simulink model "m03"  (R2019a)
settings: Solver=ode23  StartTime=0.0  StopTime=30  RelTol=1e-7
settings Model: Creator=wojta  LastModifiedBy=wojta

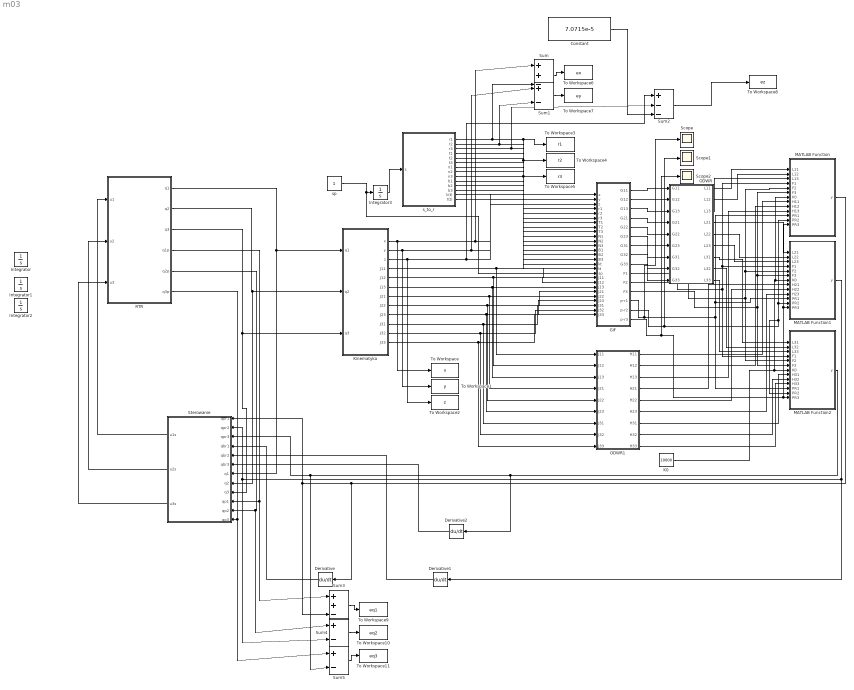
== system m03 ==
  Constant : Constant  Value=7.0715e-5
  Derivative : Derivative
  Derivative1 : Derivative
  Derivative2 : Derivative
  GiF : Subsystem
  Integrator : Integrator  InitialCondition=pi/4
  Integrator1 : Integrator  InitialCondition=0.5
  Integrator2 : Integrator  InitialCondition=-pi/2
  Integrator3 : Integrator
  K0 : Constant  Value=10000
  Kinematyka : Subsystem
  MATLAB Function : MATLAB Function  TreatAsAtomicUnit=on
  MATLAB Function1 : MATLAB Function  TreatAsAtomicUnit=on
  MATLAB Function2 : MATLAB Function  TreatAsAtomicUnit=on
  ODWR : Subsystem
  ODWR1 : Subsystem
  RTR : Subsystem
  Scope : Scope
  Scope1 : Scope
  Scope2 : Scope
  Sterowanie : Subsystem
  Sum : Sum  Inputs=|++-
  Sum1 : Sum  Inputs=|+-
  Sum2 : Sum  Inputs=|+--
  Sum3 : Sum  Inputs=|++-
  Sum4 : Sum  Inputs=|+-
  Sum5 : Sum  Inputs=|+-
  To Workspace : ToWorkspace  VariableName=x  SampleTime=-1
  To Workspace1 : ToWorkspace  VariableName=y  SampleTime=-1
  To Workspace10 : ToWorkspace  VariableName=eq2  SaveFormat=Timeseries  SampleTime=-1
  To Workspace11 : ToWorkspace  VariableName=eq3  SaveFormat=Timeseries  SampleTime=-1
  To Workspace2 : ToWorkspace  VariableName=z  SampleTime=-1
  To Workspace3 : ToWorkspace  VariableName=r1  SampleTime=-1
  To Workspace4 : ToWorkspace  VariableName=r2  SampleTime=-1
  To Workspace5 : ToWorkspace  VariableName=r3  SampleTime=-1
  To Workspace6 : ToWorkspace  VariableName=ex  SaveFormat=Timeseries  SampleTime=-1
  To Workspace7 : ToWorkspace  VariableName=ey  SaveFormat=Timeseries  SampleTime=-1
  To Workspace8 : ToWorkspace  VariableName=ez  SaveFormat=Timeseries  SampleTime=-1
  To Workspace9 : ToWorkspace  VariableName=eq1  SaveFormat=Timeseries  SampleTime=-1
  s_to_r : Subsystem
  sp : Constant
  wires:
  sp/1 -> GiF/18(sp), Integrator3/1
  Integrator3/1 -> s_to_r/1(s)
  Kinematyka/1(x) -> To Workspace/1, Sum/1, GiF/1(x)
  Kinematyka/2(y) -> To Workspace1/1, Sum1/1, GiF/2(y)
  Kinematyka/3(z) -> To Workspace2/1, Sum2/1, GiF/3(z)
  Kinematyka/4(J11) -> ODWR1/1(J11), GiF/19(J11)
  Kinematyka/5(J12) -> ODWR1/2(J12), GiF/20(J12)
  Kinematyka/6(J13) -> ODWR1/3(J13), GiF/21(J13)
  Kinematyka/7(J21) -> ODWR1/4(J21), GiF/22(J21)
  Kinematyka/8(J22) -> ODWR1/5(J22), GiF/23(J22)
  Kinematyka/9(J23) -> ODWR1/6(J23), GiF/24(J23)
  Kinematyka/10(J31) -> ODWR1/7(J31), GiF/25(J31)
  Kinematyka/11(J32) -> ODWR1/8(J32), GiF/26(J32)
  Kinematyka/12(J33) -> ODWR1/9(J33), GiF/27(J33)
  s_to_r/1(r1) -> Sum/3, To Workspace3/1, GiF/4(r1)
  s_to_r/2(r2) -> Sum1/2, To Workspace4/1, GiF/5(r2)
  s_to_r/3(r3) -> Sum2/2, To Workspace5/1, GiF/6(r3)
  s_to_r/4(t1) -> GiF/7(T1)
  s_to_r/5(t2) -> GiF/8(T2)
  s_to_r/6(t3) -> GiF/9(T3)
  s_to_r/7(n1) -> GiF/10(N1)
  s_to_r/8(n2) -> GiF/11(N2)
  s_to_r/9(n3) -> GiF/12(N3)
  s_to_r/10(b1) -> GiF/13(B1)
  s_to_r/11(b2) -> GiF/14(B2)
  s_to_r/12(b3) -> GiF/15(B3)
  s_to_r/13(k(t)) -> GiF/16(kt)
  s_to_r/14(t(t)) -> GiF/17(tt)
  GiF/1(G11) -> ODWR/1(G11)
  GiF/2(G12) -> ODWR/2(G12)
  GiF/3(G13) -> ODWR/3(G13)
  GiF/4(G21) -> ODWR/4(G21)
  GiF/5(G22) -> ODWR/5(G22)
  GiF/6(G23) -> ODWR/6(G23)
  GiF/7(G31) -> ODWR/7(G31)
  GiF/8(G32) -> ODWR/8(G32)
  GiF/9(G33) -> ODWR/9(G33)
  ODWR/1(L11) -> MATLAB Function/1(L11)
  ODWR/2(L12) -> MATLAB Function/2(L12)
  ODWR/3(L13) -> MATLAB Function/3(L13)
  ODWR/4(L21) -> MATLAB Function1/1(L21)
  ODWR/5(L22) -> MATLAB Function1/2(L22)
  ODWR/6(L23) -> MATLAB Function1/3(L23)
  ODWR/7(L31) -> MATLAB Function2/1(L31)
  ODWR/8(L32) -> MATLAB Function2/2(L32)
  ODWR/9(L33) -> MATLAB Function2/3(L33)
  GiF/10(F1) -> MATLAB Function1/4(F1), MATLAB Function/4(F1), MATLAB Function2/4(F1)
  GiF/11(F2) -> MATLAB Function1/5(F2), MATLAB Function/5(F2), MATLAB Function2/5(F2)
  GiF/12(F3) -> MATLAB Function1/6(F3), MATLAB Function/6(F3), MATLAB Function2/6(F3)
  ODWR1/1(H11) -> MATLAB Function/8(H11)
  ODWR1/2(H12) -> MATLAB Function/9(H12)
  ODWR1/3(H13) -> MATLAB Function/10(H13)
  ODWR1/4(H21) -> MATLAB Function1/8(H21)
  ODWR1/5(H22) -> MATLAB Function1/9(H22)
  ODWR1/6(H23) -> MATLAB Function1/10(H23)
  ODWR1/7(H31) -> MATLAB Function2/8(H31)
  ODWR1/8(H32) -> MATLAB Function2/9(H32)
  ODWR1/9(H33) -> MATLAB Function2/10(H33)
  GiF/13(p-r1) -> Scope/1, MATLAB Function2/11(PR1), MATLAB Function1/11(PR1), MATLAB Function/11(PR1)
  GiF/14(p-r2) -> Scope1/1, MATLAB Function2/12(PR2), MATLAB Function1/12(PR2), MATLAB Function/12(PR2)
  GiF/15(p-r3) -> Scope2/1, MATLAB Function/13(PR3), MATLAB Function1/13(PR3), MATLAB Function2/13(PR3)
  K0/1 -> MATLAB Function/7(K0), MATLAB Function1/7(K0), MATLAB Function2/7(K0)
  Sterowanie/2(u2s) -> RTR/2(u2)
  Sterowanie/1(u1s) -> RTR/1(u1)
  Sterowanie/3(u3s) -> RTR/3(u3)
  RTR/1(q1) -> Sterowanie/7(q1), Kinematyka/1(q1)
  RTR/2(q2) -> Sterowanie/8(q2), Kinematyka/2(q2)
  RTR/3(q3) -> Sterowanie/9(q3), Kinematyka/3(q3)
  Derivative/1 -> Sterowanie/4(qbr1)
  Derivative1/1 -> Sterowanie/5(qbr2)
  MATLAB Function2/1(y) -> Derivative2/1, Sum5/2, Sterowanie/3(qpr3)
  Derivative2/1 -> Sterowanie/6(qbr3)
  RTR/4(q1p) -> Sum3/1, Sterowanie/10(qp1)
  RTR/5(q2p) -> Sum4/1, Sterowanie/11(qp2)
  RTR/6(q3p) -> Sum5/1, Sterowanie/12(qp3)
  Sum/1 -> To Workspace6/1
  Sum1/1 -> To Workspace7/1
  Sum2/1 -> To Workspace8/1
  Sum5/1 -> To Workspace11/1
  Sum4/1 -> To Workspace10/1
  Sum3/1 -> To Workspace9/1
  MATLAB Function/1(y) -> Derivative/1, Sum3/3, Sterowanie/1(qpr1)
  MATLAB Function1/1(y) -> Derivative1/1, Sterowanie/2(qpr2), Sum4/2
  Constant/1 -> Sum2/3

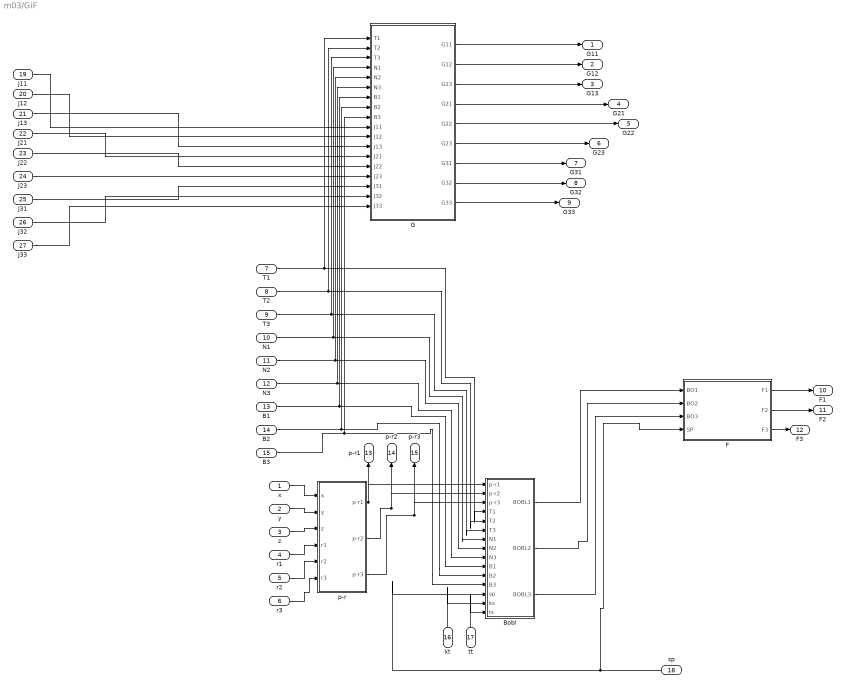
== system m03/GiF ==
  x : Inport
  y : Inport  Port=2
  z : Inport  Port=3
  r1 : Inport  Port=4
  r2 : Inport  Port=5
  r3 : Inport  Port=6
  T1 : Inport  Port=7
  T2 : Inport  Port=8
  T3 : Inport  Port=9
  N1 : Inport  Port=10
  N2 : Inport  Port=11
  N3 : Inport  Port=12
  B1 : Inport  Port=13
  B2 : Inport  Port=14
  B3 : Inport  Port=15
  kt : Inport  Port=16
  tt : Inport  Port=17
  sp : Inport  Port=18
  J11 : Inport  Port=19
  J12 : Inport  Port=20
  J13 : Inport  Port=21
  J21 : Inport  Port=22
  J22 : Inport  Port=23
  J23 : Inport  Port=24
  J31 : Inport  Port=25
  J32 : Inport  Port=26
  J33 : Inport  Port=27
  Bobl : Subsystem
  F : Subsystem
  G : Subsystem
  p-r : Subsystem
  G11 : Outport
  G12 : Outport  Port=2
  G13 : Outport  Port=3
  G21 : Outport  Port=4
  G22 : Outport  Port=5
  G23 : Outport  Port=6
  G31 : Outport  Port=7
  G32 : Outport  Port=8
  G33 : Outport  Port=9
  F1 : Outport  Port=10
  F2 : Outport  Port=11
  F3 : Outport  Port=12
  p-r1 : Outport  Port=13
  p-r2 : Outport  Port=14
  p-r3 : Outport  Port=15
  wires:
  x/1 -> p-r/1(x)
  y/1 -> p-r/2(y)
  z/1 -> p-r/3(z)
  r1/1 -> p-r/4(r1)
  r2/1 -> p-r/5(r2)
  r3/1 -> p-r/6(r3)
  p-r/1(p-r1) -> p-r1/1, Bobl/1(p-r1)
  p-r/2(p-r2) -> p-r2/1, Bobl/2(p-r2)
  p-r/3(p-r3) -> Bobl/3(p-r3), p-r3/1
  T1/1 -> G/1(T1), Bobl/4(T1)
  T2/1 -> G/2(T2), Bobl/5(T2)
  T3/1 -> G/3(T3), Bobl/6(T3)
  N1/1 -> G/4(N1), Bobl/7(N1)
  N2/1 -> G/5(N2), Bobl/8(N2)
  N3/1 -> G/6(N3), Bobl/9(N3)
  B1/1 -> G/7(B1), Bobl/10(B1)
  B2/1 -> G/8(B2), Bobl/11(B2)
  B3/1 -> G/9(B3), Bobl/12(B3)
  sp/1 -> F/4(SP), Bobl/13(sp)
  kt/1 -> Bobl/14(ks)
  tt/1 -> Bobl/15(ts)
  Bobl/1(BOBL1) -> F/1(BO1)
  Bobl/2(BOBL2) -> F/2(BO2)
  Bobl/3(BOBL3) -> F/3(BO3)
  J11/1 -> G/10(J11)
  J12/1 -> G/11(J12)
  J13/1 -> G/12(J13)
  J21/1 -> G/13(J21)
  J22/1 -> G/14(J22)
  J23/1 -> G/15(J23)
  J31/1 -> G/16(J31)
  J32/1 -> G/17(J32)
  J33/1 -> G/18(J33)
  G/1(G11) -> G11/1
  G/2(G12) -> G12/1
  G/3(G13) -> G13/1
  G/4(G21) -> G21/1
  G/5(G22) -> G22/1
  G/6(G23) -> G23/1
  G/7(G31) -> G31/1
  G/8(G32) -> G32/1
  G/9(G33) -> G33/1
  F/1(F1) -> F1/1
  F/2(F2) -> F2/1
  F/3(F3) -> F3/1

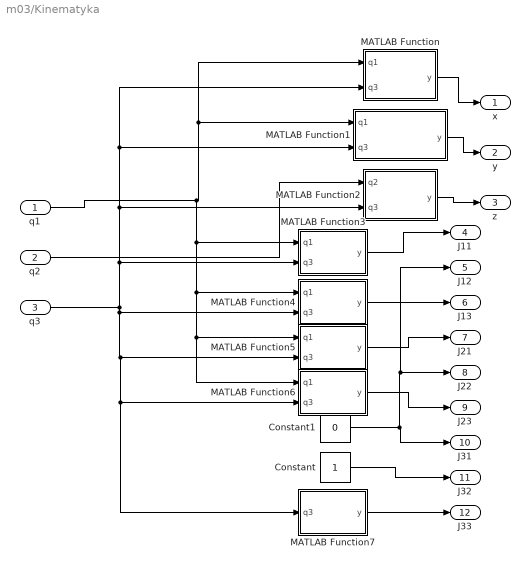
== system m03/Kinematyka ==
  q1 : Inport
  q2 : Inport  Port=2
  q3 : Inport  Port=3
  Constant : Constant
  Constant1 : Constant  Value=0
  MATLAB Function : MATLAB Function  TreatAsAtomicUnit=on
  MATLAB Function1 : MATLAB Function  TreatAsAtomicUnit=on
  MATLAB Function2 : MATLAB Function  TreatAsAtomicUnit=on
  MATLAB Function3 : MATLAB Function  TreatAsAtomicUnit=on
  MATLAB Function4 : MATLAB Function  TreatAsAtomicUnit=on
  MATLAB Function5 : MATLAB Function  TreatAsAtomicUnit=on
  MATLAB Function6 : MATLAB Function  TreatAsAtomicUnit=on
  MATLAB Function7 : MATLAB Function  TreatAsAtomicUnit=on
  x : Outport
  y : Outport  Port=2
  z : Outport  Port=3
  J11 : Outport  Port=4
  J12 : Outport  Port=5
  J13 : Outport  Port=6
  J21 : Outport  Port=7
  J22 : Outport  Port=8
  J23 : Outport  Port=9
  J31 : Outport  Port=10
  J32 : Outport  Port=11
  J33 : Outport  Port=12
  wires:
  MATLAB Function2/1(y) -> z/1
  MATLAB Function1/1(y) -> y/1
  MATLAB Function/1(y) -> x/1
  q1/1 -> MATLAB Function6/1(q1), MATLAB Function5/1(q1), MATLAB Function4/1(q1), MATLAB Function3/1(q1), MATLAB Function/1(q1), MATLAB Function1/1(q1)
  q3/1 -> MATLAB Function3/2(q3), MATLAB Function1/2(q3), MATLAB Function/2(q3), MATLAB Function2/2(q3), MATLAB Function7/1(q3), MATLAB Function6/2(q3), MATLAB Function5/2(q3), MATLAB Function4/2(q3)
  q2/1 -> MATLAB Function2/1(q2)
  MATLAB Function3/1(y) -> J11/1
  MATLAB Function4/1(y) -> J13/1
  MATLAB Function5/1(y) -> J21/1
  MATLAB Function6/1(y) -> J23/1
  MATLAB Function7/1(y) -> J33/1
  Constant/1 -> J32/1
  Constant1/1 -> J12/1, J22/1, J31/1

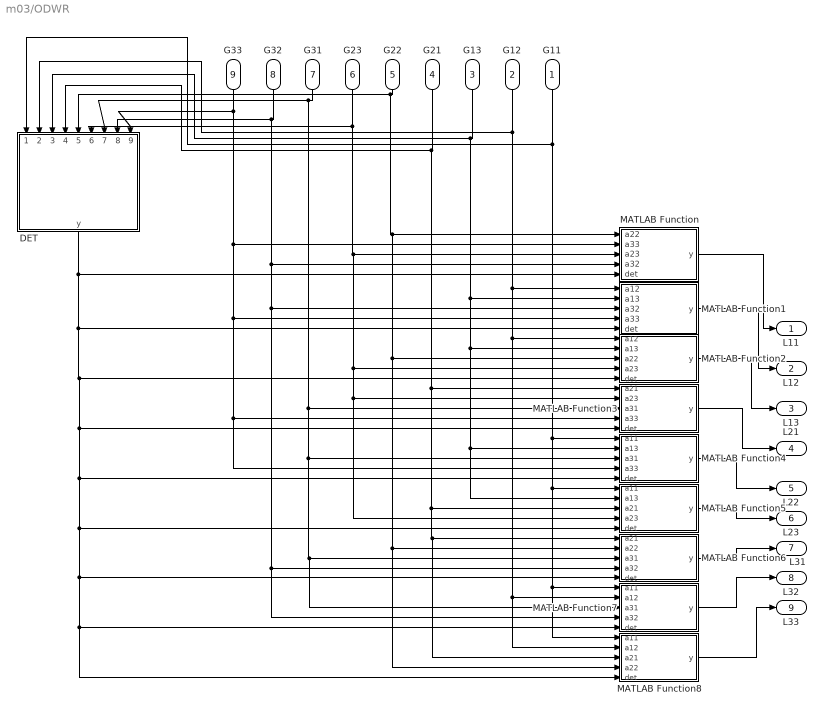
== system m03/ODWR ==
  G11 : Inport
  G12 : Inport  Port=2
  G13 : Inport  Port=3
  G21 : Inport  Port=4
  G22 : Inport  Port=5
  G23 : Inport  Port=6
  G31 : Inport  Port=7
  G32 : Inport  Port=8
  G33 : Inport  Port=9
  DET : MATLAB Function  TreatAsAtomicUnit=on
  MATLAB Function : MATLAB Function  TreatAsAtomicUnit=on
  MATLAB Function1 : MATLAB Function  TreatAsAtomicUnit=on
  MATLAB Function2 : MATLAB Function  TreatAsAtomicUnit=on
  MATLAB Function3 : MATLAB Function  TreatAsAtomicUnit=on
  MATLAB Function4 : MATLAB Function  TreatAsAtomicUnit=on
  MATLAB Function5 : MATLAB Function  TreatAsAtomicUnit=on
  MATLAB Function6 : MATLAB Function  TreatAsAtomicUnit=on
  MATLAB Function7 : MATLAB Function  TreatAsAtomicUnit=on
  MATLAB Function8 : MATLAB Function  TreatAsAtomicUnit=on
  L11 : Outport
  L12 : Outport  Port=2
  L13 : Outport  Port=3
  L21 : Outport  Port=4
  L22 : Outport  Port=5
  L23 : Outport  Port=6
  L31 : Outport  Port=7
  L32 : Outport  Port=8
  L33 : Outport  Port=9
  wires:
  MATLAB Function/1(y) -> L11/1
  MATLAB Function1/1(y) -> L12/1
  MATLAB Function2/1(y) -> L13/1
  MATLAB Function3/1(y) -> L21/1
  MATLAB Function4/1(y) -> L22/1
  MATLAB Function5/1(y) -> L23/1
  MATLAB Function6/1(y) -> L31/1
  MATLAB Function7/1(y) -> L32/1
  MATLAB Function8/1(y) -> L33/1
  G11/1 -> MATLAB Function8/1(a11), MATLAB Function7/1(a11), MATLAB Function5/1(a11), MATLAB Function4/1(a11), DET/1(a11)
  G33/1 -> MATLAB Function4/4(a33), MATLAB Function3/4(a33), MATLAB Function1/4(a33), MATLAB Function/2(a33), DET/9(a33)
  G32/1 -> MATLAB Function7/4(a32), MATLAB Function6/4(a32), MATLAB Function1/3(a32), MATLAB Function/4(a32), DET/8(a32)
  G31/1 -> MATLAB Function7/3(a31), MATLAB Function6/3(a31), MATLAB Function4/3(a31), MATLAB Function3/3(a31), DET/7(a31)
  G23/1 -> MATLAB Function5/4(a23), MATLAB Function3/2(a23), MATLAB Function2/4(a23), MATLAB Function/3(a23), DET/6(a23)
  G22/1 -> MATLAB Function8/4(a22), MATLAB Function6/2(a22), MATLAB Function2/3(a22), MATLAB Function/1(a22), DET/5(a22)
  G21/1 -> MATLAB Function8/3(a21), MATLAB Function6/1(a21), MATLAB Function5/3(a21), MATLAB Function3/1(a21), DET/4(a21)
  G13/1 -> MATLAB Function5/2(a13), MATLAB Function4/2(a13), MATLAB Function2/2(a13), MATLAB Function1/2(a13), DET/3(a13)
  G12/1 -> MATLAB Function8/2(a12), MATLAB Function7/2(a12), MATLAB Function2/1(a12), MATLAB Function1/1(a12), DET/2(a12)
  DET/1(y) -> MATLAB Function8/5(det), MATLAB Function7/5(det), MATLAB Function6/5(det), MATLAB Function5/5(det), MATLAB Function4/5(det), MATLAB Function3/5(det), MATLAB Function2/5(det), MATLAB Function1/5(det), MATLAB Function/5(det)

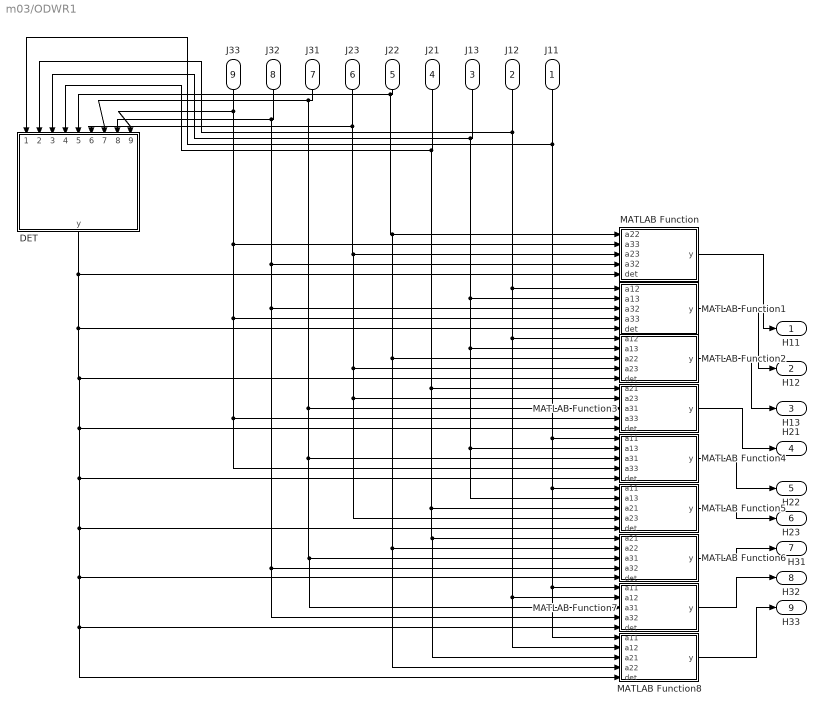
== system m03/ODWR1 ==
  J11 : Inport
  J12 : Inport  Port=2
  J13 : Inport  Port=3
  J21 : Inport  Port=4
  J22 : Inport  Port=5
  J23 : Inport  Port=6
  J31 : Inport  Port=7
  J32 : Inport  Port=8
  J33 : Inport  Port=9
  DET : MATLAB Function  TreatAsAtomicUnit=on
  MATLAB Function : MATLAB Function  TreatAsAtomicUnit=on
  MATLAB Function1 : MATLAB Function  TreatAsAtomicUnit=on
  MATLAB Function2 : MATLAB Function  TreatAsAtomicUnit=on
  MATLAB Function3 : MATLAB Function  TreatAsAtomicUnit=on
  MATLAB Function4 : MATLAB Function  TreatAsAtomicUnit=on
  MATLAB Function5 : MATLAB Function  TreatAsAtomicUnit=on
  MATLAB Function6 : MATLAB Function  TreatAsAtomicUnit=on
  MATLAB Function7 : MATLAB Function  TreatAsAtomicUnit=on
  MATLAB Function8 : MATLAB Function  TreatAsAtomicUnit=on
  H11 : Outport
  H12 : Outport  Port=2
  H13 : Outport  Port=3
  H21 : Outport  Port=4
  H22 : Outport  Port=5
  H23 : Outport  Port=6
  H31 : Outport  Port=7
  H32 : Outport  Port=8
  H33 : Outport  Port=9
  wires:
  MATLAB Function/1(y) -> H11/1
  MATLAB Function1/1(y) -> H12/1
  MATLAB Function2/1(y) -> H13/1
  MATLAB Function3/1(y) -> H21/1
  MATLAB Function4/1(y) -> H22/1
  MATLAB Function5/1(y) -> H23/1
  MATLAB Function6/1(y) -> H31/1
  MATLAB Function7/1(y) -> H32/1
  MATLAB Function8/1(y) -> H33/1
  J11/1 -> MATLAB Function8/1(a11), MATLAB Function7/1(a11), MATLAB Function5/1(a11), MATLAB Function4/1(a11), DET/1(a11)
  J33/1 -> MATLAB Function4/4(a33), MATLAB Function3/4(a33), MATLAB Function1/4(a33), MATLAB Function/2(a33), DET/9(a33)
  J32/1 -> MATLAB Function7/4(a32), MATLAB Function6/4(a32), MATLAB Function1/3(a32), MATLAB Function/4(a32), DET/8(a32)
  J31/1 -> MATLAB Function7/3(a31), MATLAB Function6/3(a31), MATLAB Function4/3(a31), MATLAB Function3/3(a31), DET/7(a31)
  J23/1 -> MATLAB Function5/4(a23), MATLAB Function3/2(a23), MATLAB Function2/4(a23), MATLAB Function/3(a23), DET/6(a23)
  J22/1 -> MATLAB Function8/4(a22), MATLAB Function6/2(a22), MATLAB Function2/3(a22), MATLAB Function/1(a22), DET/5(a22)
  J21/1 -> MATLAB Function8/3(a21), MATLAB Function6/1(a21), MATLAB Function5/3(a21), MATLAB Function3/1(a21), DET/4(a21)
  J13/1 -> MATLAB Function5/2(a13), MATLAB Function4/2(a13), MATLAB Function2/2(a13), MATLAB Function1/2(a13), DET/3(a13)
  J12/1 -> MATLAB Function8/2(a12), MATLAB Function7/2(a12), MATLAB Function2/1(a12), MATLAB Function1/1(a12), DET/2(a12)
  DET/1(y) -> MATLAB Function8/5(det), MATLAB Function7/5(det), MATLAB Function6/5(det), MATLAB Function5/5(det), MATLAB Function4/5(det), MATLAB Function3/5(det), MATLAB Function2/5(det), MATLAB Function1/5(det), MATLAB Function/5(det)

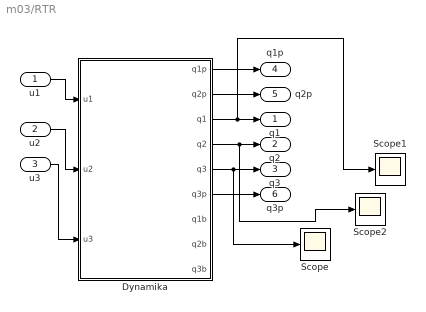
== system m03/RTR ==
  u1 : Inport
  u2 : Inport  Port=2
  u3 : Inport  Port=3
  Dynamika : Subsystem
  Scope : Scope
  Scope1 : Scope
  Scope2 : Scope
  q1 : Outport
  q2 : Outport  Port=2
  q3 : Outport  Port=3
  q1p : Outport  Port=4
  q2p : Outport  Port=5
  q3p : Outport  Port=6
  wires:
  u3/1 -> Dynamika/3(u3)
  u2/1 -> Dynamika/2(u2)
  u1/1 -> Dynamika/1(u1)
  Dynamika/3(q1) -> Scope1/1, q1/1
  Dynamika/4(q2) -> Scope2/1, q2/1
  Dynamika/5(q3) -> Scope/1, q3/1
  Dynamika/1(q1p) -> q1p/1
  Dynamika/2(q2p) -> q2p/1
  Dynamika/6(q3p) -> q3p/1

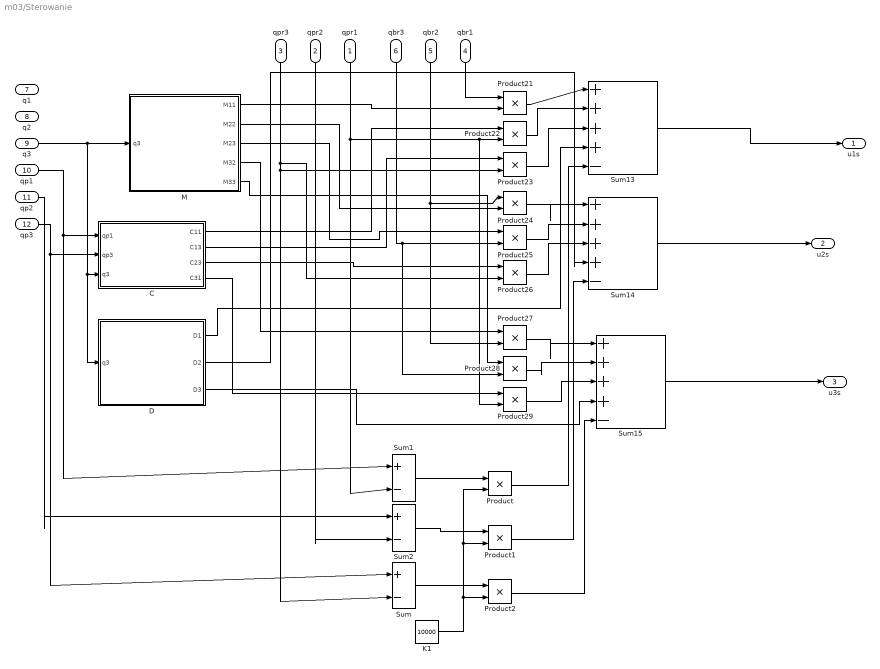
== system m03/Sterowanie ==
  qpr1 : Inport
  qpr2 : Inport  Port=2
  qpr3 : Inport  Port=3
  qbr1 : Inport  Port=4
  qbr2 : Inport  Port=5
  qbr3 : Inport  Port=6
  q1 : Inport  Port=7
  q2 : Inport  Port=8
  q3 : Inport  Port=9
  qp1 : Inport  Port=10
  qp2 : Inport  Port=11
  qp3 : Inport  Port=12
  C : Subsystem
  D : Subsystem
  K1 : Constant  Value=10000
  M : Subsystem
  Product{,1..2,21..29} (12 alike) : Product
  Sum : Sum  Inputs=|+-
  Sum1 : Sum  Inputs=|+-
  Sum13 : Sum  Inputs=|++++-
  Sum14 : Sum  Inputs=|++++-
  Sum15 : Sum  Inputs=|++++-
  Sum2 : Sum  Inputs=|+-
  u1s : Outport
  u2s : Outport  Port=2
  u3s : Outport  Port=3
  wires:
  Sum14/1 -> u2s/1
  Sum15/1 -> u3s/1
  Sum13/1 -> u1s/1
  Product21/1 -> Sum13/1
  Product22/1 -> Sum13/2
  Product23/1 -> Sum13/3
  Product24/1 -> Sum14/1
  Product25/1 -> Sum14/2
  Product26/1 -> Sum14/3
  Product27/1 -> Sum15/1
  Product28/1 -> Sum15/2
  Product29/1 -> Sum15/3
  q3/1 -> D/1(q3), C/3(q3), M/1(q3)
  qp1/1 -> Sum1/1, C/1(qp1)
  qp3/1 -> Sum/1, C/2(qp3)
  qbr1/1 -> Product21/1
  M/1(M11) -> Product21/2
  C/1(C11) -> Product22/1
  C/2(C13) -> Product23/1
  C/3(C23) -> Product26/1
  M/2(M22) -> Product24/2
  M/3(M23) -> Product25/1
  D/1(D1) -> Sum13/4
  D/2(D2) -> Sum14/4
  D/3(D3) -> Sum15/4
  M/4(M32) -> Product27/1
  M/5(M33) -> Product28/1
  C/4(C31) -> Product29/1
  qpr1/1 -> Sum1/2, Product29/2, Product22/2
  qpr3/1 -> Product23/2, Sum/2, Product26/2
  qbr2/1 -> Product27/2, Product24/1
  qbr3/1 -> Product25/2, Product28/2
  qp2/1 -> Sum2/1
  qpr2/1 -> Sum2/2
  K1/1 -> Product/2, Product1/2, Product2/2
  Sum2/1 -> Product1/1
  Sum/1 -> Product2/1
  Sum1/1 -> Product/1
  Product/1 -> Sum13/5
  Product1/1 -> Sum14/5
  Product2/1 -> Sum15/5

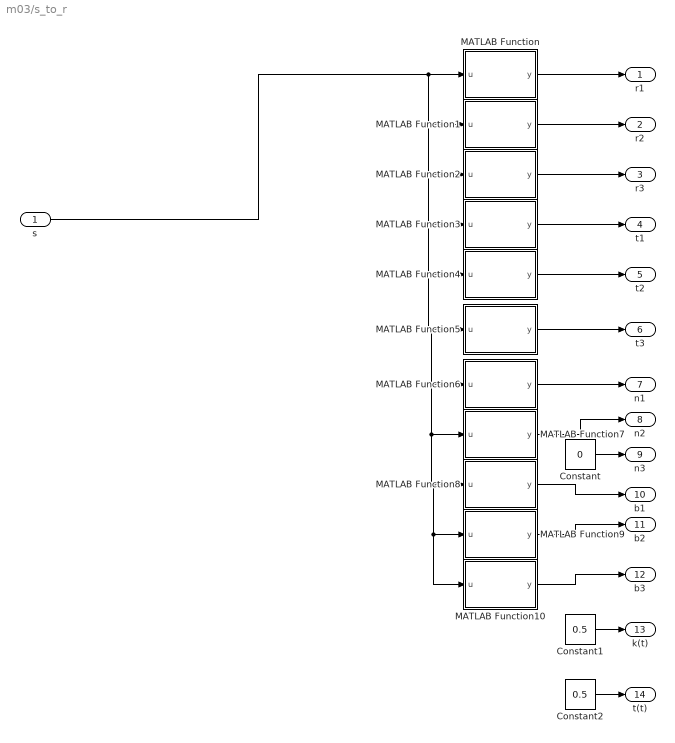
== system m03/s_to_r ==
  s : Inport
  Constant : Constant  Value=0
  Constant1 : Constant  Value=0.5
  Constant2 : Constant  Value=0.5
  MATLAB Function : MATLAB Function  TreatAsAtomicUnit=on
  MATLAB Function1 : MATLAB Function  TreatAsAtomicUnit=on
  MATLAB Function10 : MATLAB Function  TreatAsAtomicUnit=on
  MATLAB Function2 : MATLAB Function  TreatAsAtomicUnit=on
  MATLAB Function3 : MATLAB Function  TreatAsAtomicUnit=on
  MATLAB Function4 : MATLAB Function  TreatAsAtomicUnit=on
  MATLAB Function5 : MATLAB Function  TreatAsAtomicUnit=on
  MATLAB Function6 : MATLAB Function  TreatAsAtomicUnit=on
  MATLAB Function7 : MATLAB Function  TreatAsAtomicUnit=on
  MATLAB Function8 : MATLAB Function  TreatAsAtomicUnit=on
  MATLAB Function9 : MATLAB Function  TreatAsAtomicUnit=on
  r1 : Outport
  r2 : Outport  Port=2
  r3 : Outport  Port=3
  t1 : Outport  Port=4
  t2 : Outport  Port=5
  t3 : Outport  Port=6
  n1 : Outport  Port=7
  n2 : Outport  Port=8
  n3 : Outport  Port=9
  b1 : Outport  Port=10
  b2 : Outport  Port=11
  b3 : Outport  Port=12
  k(t) : Outport  Port=13
  t(t) : Outport  Port=14
  wires:
  MATLAB Function/1(y) -> r1/1
  MATLAB Function1/1(y) -> r2/1
  MATLAB Function2/1(y) -> r3/1
  MATLAB Function3/1(y) -> t1/1
  MATLAB Function4/1(y) -> t2/1
  MATLAB Function5/1(y) -> t3/1
  MATLAB Function6/1(y) -> n1/1
  MATLAB Function7/1(y) -> n2/1
  Constant/1 -> n3/1
  MATLAB Function8/1(y) -> b1/1
  MATLAB Function9/1(y) -> b2/1
  MATLAB Function10/1(y) -> b3/1
  Constant1/1 -> k(t)/1
  Constant2/1 -> t(t)/1
  s/1 -> MATLAB Function10/1(u), MATLAB Function9/1(u), MATLAB Function8/1(u), MATLAB Function7/1(u), MATLAB Function6/1(u), MATLAB Function5/1(u), MATLAB Function4/1(u), MATLAB Function3/1(u), MATLAB Function2/1(u), MATLAB Function1/1(u), MATLAB Function/1(u)

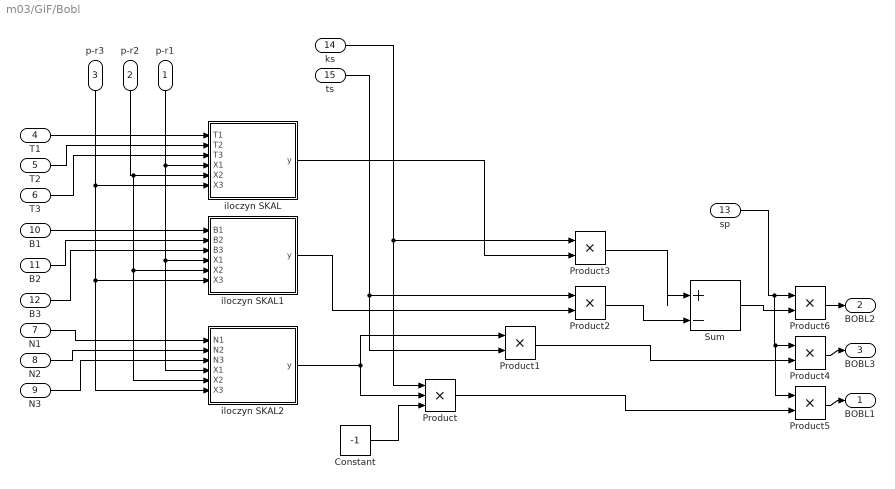
== system m03/GiF/Bobl ==
  p-r1 : Inport
  p-r2 : Inport  Port=2
  p-r3 : Inport  Port=3
  T1 : Inport  Port=4
  T2 : Inport  Port=5
  T3 : Inport  Port=6
  N1 : Inport  Port=7
  N2 : Inport  Port=8
  N3 : Inport  Port=9
  B1 : Inport  Port=10
  B2 : Inport  Port=11
  B3 : Inport  Port=12
  sp : Inport  Port=13
  ks : Inport  Port=14
  ts : Inport  Port=15
  Constant : Constant  Value=-1
  Product : Product  Inputs=3
  Product{1..6} (6 alike) : Product
  Sum : Sum  Inputs=|+-
  iloczyn SKAL : MATLAB Function  TreatAsAtomicUnit=on
  iloczyn SKAL1 : MATLAB Function  TreatAsAtomicUnit=on
  iloczyn SKAL2 : MATLAB Function  TreatAsAtomicUnit=on
  BOBL1 : Outport
  BOBL2 : Outport  Port=2
  BOBL3 : Outport  Port=3
  wires:
  T1/1 -> iloczyn SKAL/1(T1)
  T2/1 -> iloczyn SKAL/2(T2)
  T3/1 -> iloczyn SKAL/3(T3)
  B1/1 -> iloczyn SKAL1/1(B1)
  B2/1 -> iloczyn SKAL1/2(B2)
  B3/1 -> iloczyn SKAL1/3(B3)
  N1/1 -> iloczyn SKAL2/1(N1)
  N2/1 -> iloczyn SKAL2/2(N2)
  N3/1 -> iloczyn SKAL2/3(N3)
  p-r2/1 -> iloczyn SKAL2/5(X2), iloczyn SKAL1/5(X2), iloczyn SKAL/5(X2)
  p-r3/1 -> iloczyn SKAL1/6(X3), iloczyn SKAL2/6(X3), iloczyn SKAL/6(X3)
  p-r1/1 -> iloczyn SKAL2/4(X1), iloczyn SKAL1/4(X1), iloczyn SKAL/4(X1)
  Constant/1 -> Product/3
  iloczyn SKAL2/1(y) -> Product/2, Product1/1
  ks/1 -> Product3/1, Product/1
  ts/1 -> Product2/1, Product1/2
  Product2/1 -> Sum/2
  Product3/1 -> Sum/1
  iloczyn SKAL/1(y) -> Product3/2
  iloczyn SKAL1/1(y) -> Product2/2
  Product6/1 -> BOBL2/1
  Sum/1 -> Product6/2
  Product4/1 -> BOBL3/1
  Product1/1 -> Product4/2
  Product5/1 -> BOBL1/1
  Product/1 -> Product5/2
  sp/1 -> Product5/1, Product4/1, Product6/1

== system m03/GiF/F ==
  BO1 : Inport
  BO2 : Inport  Port=2
  BO3 : Inport  Port=3
  SP : Inport  Port=4
  Sum : Sum  Inputs=|--
  Sum1 : Sum  Inputs=|--
  Sum2 : Sum  Inputs=|--
  F1 : Outport
  F2 : Outport  Port=2
  F3 : Outport  Port=3
  wires:
  BO1/1 -> Sum/1
  BO2/1 -> Sum1/1
  BO3/1 -> Sum2/1
  SP/1 -> Sum2/2, Sum/2, Sum1/2
  Sum/1 -> F1/1
  Sum1/1 -> F2/1
  Sum2/1 -> F3/1

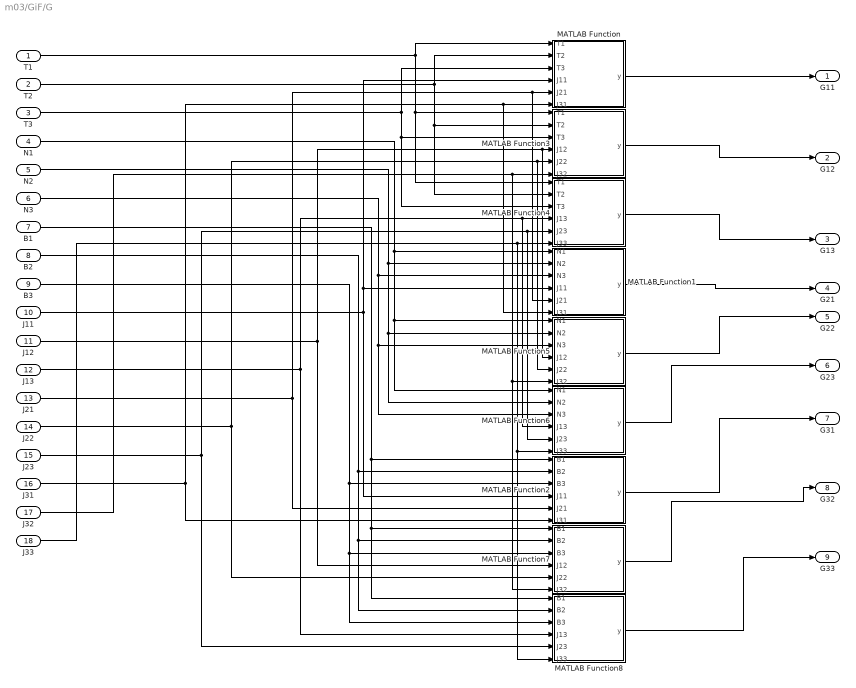
== system m03/GiF/G ==
  T1 : Inport
  T2 : Inport  Port=2
  T3 : Inport  Port=3
  N1 : Inport  Port=4
  N2 : Inport  Port=5
  N3 : Inport  Port=6
  B1 : Inport  Port=7
  B2 : Inport  Port=8
  B3 : Inport  Port=9
  J11 : Inport  Port=10
  J12 : Inport  Port=11
  J13 : Inport  Port=12
  J21 : Inport  Port=13
  J22 : Inport  Port=14
  J23 : Inport  Port=15
  J31 : Inport  Port=16
  J32 : Inport  Port=17
  J33 : Inport  Port=18
  MATLAB Function : MATLAB Function  TreatAsAtomicUnit=on
  MATLAB Function1 : MATLAB Function  TreatAsAtomicUnit=on
  MATLAB Function2 : MATLAB Function  TreatAsAtomicUnit=on
  MATLAB Function3 : MATLAB Function  TreatAsAtomicUnit=on
  MATLAB Function4 : MATLAB Function  TreatAsAtomicUnit=on
  MATLAB Function5 : MATLAB Function  TreatAsAtomicUnit=on
  MATLAB Function6 : MATLAB Function  TreatAsAtomicUnit=on
  MATLAB Function7 : MATLAB Function  TreatAsAtomicUnit=on
  MATLAB Function8 : MATLAB Function  TreatAsAtomicUnit=on
  G11 : Outport
  G12 : Outport  Port=2
  G13 : Outport  Port=3
  G21 : Outport  Port=4
  G22 : Outport  Port=5
  G23 : Outport  Port=6
  G31 : Outport  Port=7
  G32 : Outport  Port=8
  G33 : Outport  Port=9
  wires:
  MATLAB Function/1(y) -> G11/1
  MATLAB Function1/1(y) -> G21/1
  MATLAB Function2/1(y) -> G31/1
  MATLAB Function3/1(y) -> G12/1
  MATLAB Function4/1(y) -> G13/1
  MATLAB Function5/1(y) -> G22/1
  MATLAB Function6/1(y) -> G23/1
  MATLAB Function7/1(y) -> G32/1
  MATLAB Function8/1(y) -> G33/1
  T1/1 -> MATLAB Function/1(T1), MATLAB Function4/1(T1), MATLAB Function3/1(T1)
  T2/1 -> MATLAB Function/2(T2), MATLAB Function4/2(T2), MATLAB Function3/2(T2)
  T3/1 -> MATLAB Function/3(T3), MATLAB Function3/3(T3), MATLAB Function4/3(T3)
  N1/1 -> MATLAB Function6/1(N1), MATLAB Function5/1(N1), MATLAB Function1/1(N1)
  N2/1 -> MATLAB Function6/2(N2), MATLAB Function5/2(N2), MATLAB Function1/2(N2)
  N3/1 -> MATLAB Function6/3(N3), MATLAB Function5/3(N3), MATLAB Function1/3(N3)
  B1/1 -> MATLAB Function8/1(B1), MATLAB Function7/1(B1), MATLAB Function2/1(B1)
  B2/1 -> MATLAB Function8/2(B2), MATLAB Function7/2(B2), MATLAB Function2/2(B2)
  B3/1 -> MATLAB Function8/3(B3), MATLAB Function7/3(B3), MATLAB Function2/3(B3)
  J11/1 -> MATLAB Function1/4(J11), MATLAB Function/4(J11), MATLAB Function2/4(J11)
  J12/1 -> MATLAB Function5/4(J12), MATLAB Function3/4(J12), MATLAB Function7/4(J12)
  J13/1 -> MATLAB Function4/4(J13), MATLAB Function6/4(J13), MATLAB Function8/4(J13)
  J21/1 -> MATLAB Function/5(J21), MATLAB Function1/5(J21), MATLAB Function2/5(J21)
  J22/1 -> MATLAB Function7/5(J22), MATLAB Function3/5(J22), MATLAB Function5/5(J22)
  J23/1 -> MATLAB Function8/5(J23), MATLAB Function4/5(J23), MATLAB Function6/5(J23)
  J31/1 -> MATLAB Function2/6(J31), MATLAB Function/6(J31), MATLAB Function1/6(J31)
  J32/1 -> MATLAB Function5/6(J32), MATLAB Function7/6(J32), MATLAB Function3/6(J32)
  J33/1 -> MATLAB Function6/6(J33), MATLAB Function8/6(J33), MATLAB Function4/6(J33)

== system m03/GiF/p-r ==
  x : Inport
  y : Inport  Port=2
  z : Inport  Port=3
  r1 : Inport  Port=4
  r2 : Inport  Port=5
  r3 : Inport  Port=6
  Sum : Sum  Inputs=|+-
  Sum1 : Sum  Inputs=|+-
  Sum2 : Sum  Inputs=|+-
  p-r1 : Outport
  p-r2 : Outport  Port=2
  p-r3 : Outport  Port=3
  wires:
  Sum/1 -> p-r1/1
  Sum2/1 -> p-r3/1
  Sum1/1 -> p-r2/1
  x/1 -> Sum/1
  y/1 -> Sum1/1
  z/1 -> Sum2/1
  r1/1 -> Sum/2
  r2/1 -> Sum1/2
  r3/1 -> Sum2/2

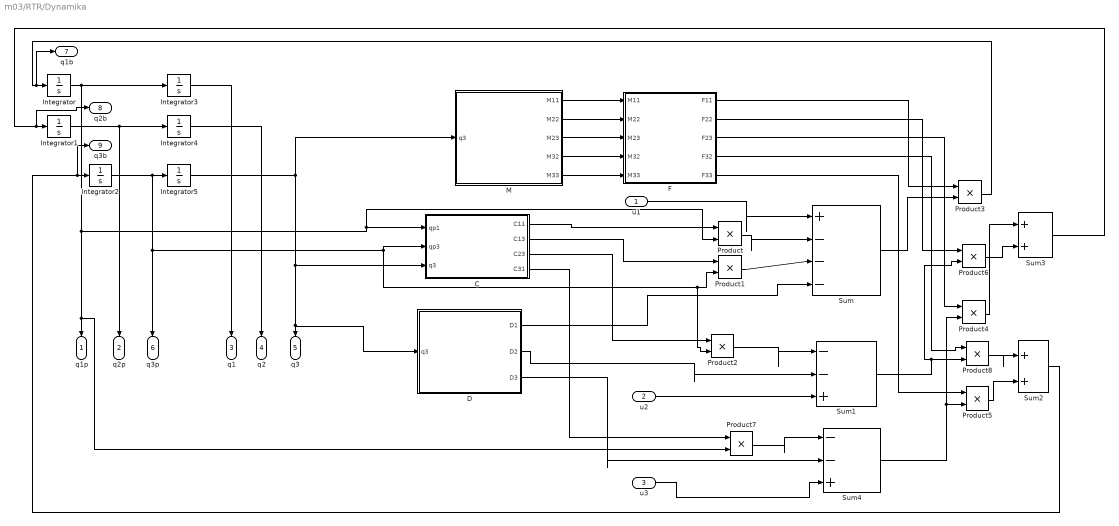
== system m03/RTR/Dynamika ==
  u1 : Inport
  u2 : Inport  Port=2
  u3 : Inport  Port=3
  C : Subsystem
  D : Subsystem
  F : Subsystem
  Integrator : Integrator
  Integrator1 : Integrator
  Integrator2 : Integrator
  Integrator3 : Integrator  InitialCondition=pi/4
  Integrator4 : Integrator  InitialCondition=0.5
  Integrator5 : Integrator  InitialCondition=-pi/2
  M : Subsystem
  Product{,1..8} (9 alike) : Product
  Sum : Sum  Inputs=|+---
  Sum1 : Sum  Inputs=|--+
  Sum2 : Sum  Inputs=|++
  Sum3 : Sum  Inputs=|++
  Sum4 : Sum  Inputs=|--+
  q1p : Outport
  q2p : Outport  Port=2
  q1 : Outport  Port=3
  q2 : Outport  Port=4
  q3 : Outport  Port=5
  q3p : Outport  Port=6
  q1b : Outport  Port=7
  q2b : Outport  Port=8
  q3b : Outport  Port=9
  wires:
  Product6/1 -> Sum3/2
  Sum3/1 -> q2b/1, Integrator1/1
  Integrator1/1 -> Integrator4/1, q2p/1
  Integrator4/1 -> q2/1
  D/2(D2) -> Sum1/2
  C/1(C11) -> Product/1
  D/1(D1) -> Sum/4
  C/3(C23) -> Product2/1
  C/2(C13) -> Product1/1
  Sum/1 -> Product3/2
  M/2(M22) -> F/2(M22)
  M/1(M11) -> F/1(M11)
  M/4(M32) -> F/4(M32)
  Product2/1 -> Sum1/1
  Product1/1 -> Sum/3
  M/3(M23) -> F/3(M23)
  u2/1 -> Sum1/3
  Product/1 -> Sum/2
  Integrator3/1 -> q1/1
  u1/1 -> Sum/1
  Integrator2/1 -> Integrator5/1, q3p/1, Product2/2, Product1/2, C/2(qp3)
  Integrator5/1 -> D/1(q3), q3/1, C/3(q3), M/1(q3)
  M/5(M33) -> F/5(M33)
  Integrator/1 -> Integrator3/1, Product7/2, q1p/1, Product/2, C/1(qp1)
  u3/1 -> Sum4/3
  D/3(D3) -> Sum4/2
  Product7/1 -> Sum4/1
  C/4(C31) -> Product7/1
  F/1(F11) -> Product3/1
  Product3/1 -> q1b/1, Integrator/1
  Sum1/1 -> Product8/2, Product6/2
  Sum4/1 -> Product5/2, Product4/2
  F/2(F22) -> Product6/1
  F/3(F23) -> Product4/1
  Product4/1 -> Sum3/1
  F/4(F32) -> Product8/1
  Product8/1 -> Sum2/1
  Product5/1 -> Sum2/2
  F/5(F33) -> Product5/1
  Sum2/1 -> q3b/1, Integrator2/1

== system m03/Sterowanie/C ==
  qp1 : Inport
  qp3 : Inport  Port=2
  q3 : Inport  Port=3
  MATLAB Function : MATLAB Function  TreatAsAtomicUnit=on
  MATLAB Function1 : MATLAB Function  TreatAsAtomicUnit=on
  MATLAB Function2 : MATLAB Function  TreatAsAtomicUnit=on
  MATLAB Function3 : MATLAB Function  TreatAsAtomicUnit=on
  C11 : Outport
  C13 : Outport  Port=2
  C23 : Outport  Port=3
  C31 : Outport  Port=4
  wires:
  MATLAB Function/1(y) -> C11/1
  MATLAB Function1/1(y) -> C13/1
  MATLAB Function2/1(y) -> C23/1
  MATLAB Function3/1(y) -> C31/1
  qp3/1 -> MATLAB Function2/2(qp3), MATLAB Function/2(qp3)
  q3/1 -> MATLAB Function1/2(q3), MATLAB Function/1(q3), MATLAB Function3/1(q3), MATLAB Function2/1(q3)
  qp1/1 -> MATLAB Function3/2(qp1), MATLAB Function1/1(qp1)

== system m03/Sterowanie/D ==
  q3 : Inport
  Constant : Constant  Value=0
  Constant1 : Constant  Value=392.4
  MATLAB Function : MATLAB Function  TreatAsAtomicUnit=on
  D1 : Outport
  D2 : Outport  Port=2
  D3 : Outport  Port=3
  wires:
  Constant/1 -> D1/1
  Constant1/1 -> D2/1
  MATLAB Function/1(y) -> D3/1
  q3/1 -> MATLAB Function/1(q3)

== system m03/Sterowanie/M ==
  q3 : Inport
  Constant : Constant  Value=40
  Constant1 : Constant  Value=4/15
  MATLAB Function : MATLAB Function  TreatAsAtomicUnit=on
  MATLAB Function2 : MATLAB Function  TreatAsAtomicUnit=on
  MATLAB Function3 : MATLAB Function  TreatAsAtomicUnit=on
  M11 : Outport
  M22 : Outport  Port=2
  M23 : Outport  Port=3
  M32 : Outport  Port=4
  M33 : Outport  Port=5
  wires:
  q3/1 -> MATLAB Function3/1(u), MATLAB Function2/1(u), MATLAB Function/1(u)
  MATLAB Function/1(y) -> M11/1
  Constant/1 -> M22/1
  MATLAB Function2/1(y) -> M23/1
  MATLAB Function3/1(y) -> M32/1
  Constant1/1 -> M33/1

== system m03/RTR/Dynamika/C ==
  qp1 : Inport
  qp3 : Inport  Port=2
  q3 : Inport  Port=3
  MATLAB Function : MATLAB Function  TreatAsAtomicUnit=on
  MATLAB Function1 : MATLAB Function  TreatAsAtomicUnit=on
  MATLAB Function2 : MATLAB Function  TreatAsAtomicUnit=on
  MATLAB Function3 : MATLAB Function  TreatAsAtomicUnit=on
  C11 : Outport
  C13 : Outport  Port=2
  C23 : Outport  Port=3
  C31 : Outport  Port=4
  wires:
  MATLAB Function/1(y) -> C11/1
  MATLAB Function1/1(y) -> C13/1
  MATLAB Function2/1(y) -> C23/1
  MATLAB Function3/1(y) -> C31/1
  qp3/1 -> MATLAB Function2/2(qp3), MATLAB Function/2(qp3)
  q3/1 -> MATLAB Function1/2(q3), MATLAB Function/1(q3), MATLAB Function3/1(q3), MATLAB Function2/1(q3)
  qp1/1 -> MATLAB Function3/2(qp1), MATLAB Function1/1(qp1)

== system m03/RTR/Dynamika/D ==
  q3 : Inport
  Constant : Constant  Value=0
  Constant1 : Constant  Value=392.4
  MATLAB Function : MATLAB Function  TreatAsAtomicUnit=on
  D1 : Outport
  D2 : Outport  Port=2
  D3 : Outport  Port=3
  wires:
  Constant/1 -> D1/1
  Constant1/1 -> D2/1
  MATLAB Function/1(y) -> D3/1
  q3/1 -> MATLAB Function/1(q3)

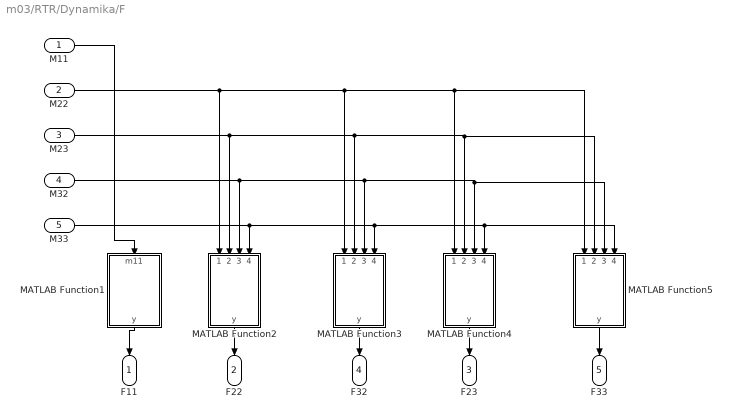
== system m03/RTR/Dynamika/F ==
  M11 : Inport
  M22 : Inport  Port=2
  M23 : Inport  Port=3
  M32 : Inport  Port=4
  M33 : Inport  Port=5
  MATLAB Function1 : MATLAB Function  TreatAsAtomicUnit=on
  MATLAB Function2 : MATLAB Function  TreatAsAtomicUnit=on
  MATLAB Function3 : MATLAB Function  TreatAsAtomicUnit=on
  MATLAB Function4 : MATLAB Function  TreatAsAtomicUnit=on
  MATLAB Function5 : MATLAB Function  TreatAsAtomicUnit=on
  F11 : Outport
  F22 : Outport  Port=2
  F23 : Outport  Port=3
  F32 : Outport  Port=4
  F33 : Outport  Port=5
  wires:
  MATLAB Function1/1(y) -> F11/1
  MATLAB Function2/1(y) -> F22/1
  M11/1 -> MATLAB Function1/1(m11)
  MATLAB Function5/1(y) -> F33/1
  M23/1 -> MATLAB Function5/2(m23), MATLAB Function4/2(m23), MATLAB Function3/2(m23), MATLAB Function2/2(m23)
  M32/1 -> MATLAB Function5/3(m32), MATLAB Function4/3(m32), MATLAB Function3/3(m32), MATLAB Function2/3(m32)
  M33/1 -> MATLAB Function5/4(m33), MATLAB Function4/4(m33), MATLAB Function3/4(m33), MATLAB Function2/4(m33)
  M22/1 -> MATLAB Function5/1(m22), MATLAB Function4/1(m22), MATLAB Function3/1(m22), MATLAB Function2/1(m22)
  MATLAB Function3/1(y) -> F32/1
  MATLAB Function4/1(y) -> F23/1

== system m03/RTR/Dynamika/M ==
  q3 : Inport
  Constant : Constant  Value=40
  Constant1 : Constant  Value=4/15
  MATLAB Function : MATLAB Function  TreatAsAtomicUnit=on
  MATLAB Function2 : MATLAB Function  TreatAsAtomicUnit=on
  MATLAB Function3 : MATLAB Function  TreatAsAtomicUnit=on
  M11 : Outport
  M22 : Outport  Port=2
  M23 : Outport  Port=3
  M32 : Outport  Port=4
  M33 : Outport  Port=5
  wires:
  q3/1 -> MATLAB Function3/1(u), MATLAB Function2/1(u), MATLAB Function/1(u)
  MATLAB Function/1(y) -> M11/1
  Constant/1 -> M22/1
  MATLAB Function2/1(y) -> M23/1
  MATLAB Function3/1(y) -> M32/1
  Constant1/1 -> M33/1

== matlab function m03/s_to_r/MATLAB Function1 ==
  data: u input; y output
function y = fcn(u)

y = sin(u/sqrt(2));

== matlab function m03/s_to_r/MATLAB Function ==
  data: u input; y output
function y = fcn(u)

y = cos(u/sqrt(2));

== matlab function m03/s_to_r/MATLAB Function2 ==
  data: u input; y output
function y = fcn(u)

y = u/sqrt(2);

== matlab function m03/s_to_r/MATLAB Function3 ==
  data: u input; y output
function y = fcn(u)

y = (-sin(u/sqrt(2)))/sqrt(2);

== matlab function m03/s_to_r/MATLAB Function4 ==
  data: u input; y output
function y = fcn(u)

y = (cos(u/sqrt(2)))/sqrt(2);

== matlab function m03/s_to_r/MATLAB Function5 ==
  data: u input; y output
function y = fcn(u)

y = 1/sqrt(2);

== matlab function m03/s_to_r/MATLAB Function6 ==
  data: u input; y output
function y = fcn(u)

y = -cos(u/sqrt(2));

== matlab function m03/s_to_r/MATLAB Function7 ==
  data: u input; y output
function y = fcn(u)

y = -sin(u/sqrt(2));

== matlab function m03/s_to_r/MATLAB Function8 ==
  data: u input; y output
function y = fcn(u)

y = (sin(u/sqrt(2)))/sqrt(2);

== matlab function m03/s_to_r/MATLAB Function9 ==
  data: u input; y output
function y = fcn(u)

y = (-cos(u/sqrt(2)))/sqrt(2);

== matlab function m03/s_to_r/MATLAB Function10 ==
  data: u input; y output
function y = fcn(u)

y = 1/sqrt(2);

== matlab function m03/ODWR1/DET ==
  data: a11 input; y output; a12 input; a13 input; a21 input; a22 input; a23 input; a31 input; a32 input; a33 input
function y = fcn(a11, a12, a13, a21, a22, a23, a31, a32, a33)

y = a11*a22*a33+a21*a32*a13+a31*a12*a23-a11*a32*a23-a31*a22*a13-a21*a12*a33;

== matlab function m03/ODWR1/MATLAB Function ==
  data: a22 input; y output; a33 input; a23 input; a32 input; det input
function y = fcn(a22, a33, a23, a32, det)

y = (a22*a33-a23*a32)/det;

== matlab function m03/ODWR1/MATLAB Function1 ==
  data: a12 input; a13 input; a32 input; y output; a33 input; det input
function y = fcn(a12, a13, a32, a33, det)

y = (a13*a32-a12*a33)/det;

== matlab function m03/ODWR1/MATLAB Function2 ==
  data: a12 input; a13 input; a22 input; y output; a23 input; det input
function y = fcn(a12, a13, a22, a23, det)

y = (a12*a23-a13*a22)/det;

== matlab function m03/ODWR1/MATLAB Function3 ==
  data: a21 input; a23 input; a31 input; y output; a33 input; det input
function y = fcn(a21, a23, a31, a33, det)

y = (a23*a31-a21*a33)/det;

== matlab function m03/ODWR1/MATLAB Function4 ==
  data: a11 input; a13 input; a31 input; y output; a33 input; det input
function y = fcn(a11, a13, a31, a33, det)

y = (a11*a33-a13*a31)/det;

== matlab function m03/ODWR1/MATLAB Function5 ==
  data: a11 input; y output; a13 input; a21 input; a23 input; det input
function y = fcn(a11, a13, a21, a23, det)

y = (a13*a21-a11*a23)/det;

== matlab function m03/ODWR1/MATLAB Function6 ==
  data: a21 input; a22 input; y output; a31 input; a32 input; det input
function y = fcn(a21, a22, a31, a32, det)

y = (a21*a32-a22*a31)/det;

== matlab function m03/ODWR1/MATLAB Function7 ==
  data: a11 input; y output; a12 input; a31 input; a32 input; det input
function y = fcn(a11, a12, a31, a32, det)

y = (a12*a31-a11*a32)/det;

== matlab function m03/ODWR1/MATLAB Function8 ==
  data: a11 input; a12 input; a21 input; a22 input; y output; det input
function y = fcn(a11, a12, a21, a22, det)

y = (a11*a22-a12*a21)/det;

== matlab function m03/MATLAB Function ==
  data: L11 input; y output; L12 input; L13 input; F1 input; F2 input; F3 input; K0 input; H11 input; H12 input; H13 input; PR1 input; PR2 input; PR3 input
function y = fcn(L11, L12, L13, F1, F2, F3, K0, H11, H12, H13, PR1, PR2, PR3)

y = -(L11*F1+ L12*F2+ L13*F3)-K0*(H11*PR1+ H12*PR2+ H13*PR3);

== matlab function m03/MATLAB Function1 ==
  data: L21 input; y output; L22 input; L23 input; F1 input; F2 input; F3 input; K0 input; H21 input; H22 input; H23 input; PR1 input; PR2 input; PR3 input
function y = fcn(L21, L22, L23, F1, F2, F3, K0, H21, H22, H23, PR1, PR2, PR3)

y = -(L21*F1+ L22*F2+ L23*F3)-K0*(H21*PR1+ H22*PR2+ H23*PR3);

== matlab function m03/MATLAB Function2 ==
  data: L31 input; y output; L32 input; L33 input; F1 input; F2 input; F3 input; K0 input; H31 input; H32 input; H33 input; PR1 input; PR2 input; PR3 input
function y = fcn(L31, L32, L33, F1, F2, F3, K0, H31, H32, H33, PR1, PR2, PR3)

y = -(L31*F1+ L32*F2+ L33*F3)-K0*(H31*PR1+ H32*PR2+ H33*PR3);

== matlab function m03/Sterowanie/C/MATLAB Function ==
  data: q3 input; y output; qp3 input
function y = fcn(q3, qp3)
%#codegen

y =qp3*(-0.6*sin(q3)-(4/15)*sin(q3)*cos(q3));

== matlab function m03/Sterowanie/C/MATLAB Function1 ==
  data: qp1 input; y output; q3 input
function y = fcn(qp1,q3)
%#codegen

y = -qp1*(0.6*sin(q3)+(4/15)*sin(q3)*cos(q3));

== matlab function m03/Sterowanie/C/MATLAB Function2 ==
  data: q3 input; y output; qp3 input
function y = fcn(q3, qp3)
%#codegen

y = -qp3*0.6*sin(q3);

== matlab function m03/Sterowanie/C/MATLAB Function3 ==
  data: q3 input; y output; qp1 input
function y = fcn(q3, qp1)
%#codegen

y = qp1*(0.6*sin(q3)+(4/15)*sin(q3)*cos(q3));

== matlab function m03/Sterowanie/D/MATLAB Function ==
  data: q3 input; y output
function y = fcn(q3)
%#codegen

y = 0.5*9.81*20*0.2*cos(q3);

== matlab function m03/Sterowanie/M/MATLAB Function ==
  data: u input; y output
function y = fcn(u)
%#codegen

y = 0.6 +1.8+(4/15)*(cos(u)*cos(u))+1.2*cos(u);

== matlab function m03/Sterowanie/M/MATLAB Function2 ==
  data: u input; y output
function y = fcn(u)
%#codegen

y = 0.6*cos(u);

== matlab function m03/Sterowanie/M/MATLAB Function3 ==
  data: u input; y output
function y = fcn(u)
%#codegen

y = 0.6*cos(u);

== matlab function m03/GiF/Bobl/iloczyn SKAL ==
  data: T1 input; y output; T2 input; T3 input; X1 input; X2 input; X3 input
function y = fcn(T1, T2, T3, X1,X2, X3)

y = T1*X1+T2*X2+T3*X3;

== matlab function m03/GiF/Bobl/iloczyn SKAL1 ==
  data: B1 input; y output; B2 input; B3 input; X1 input; X2 input; X3 input
function y = fcn(B1, B2, B3, X1,X2, X3)

y = B1*X1+B2*X2+B3*X3;

== matlab function m03/GiF/Bobl/iloczyn SKAL2 ==
  data: N1 input; y output; N2 input; N3 input; X1 input; X2 input; X3 input
function y = fcn(N1, N2, N3, X1,X2, X3)

y = N1*X1+N2*X2+N3*X3;

== matlab function m03/GiF/G/MATLAB Function ==
  data: T1 input; y output; T2 input; T3 input; J11 input; J21 input; J31 input
function y = fcn(T1, T2, T3, J11, J21, J31)

y = T1*J11+T2*J21+T3*J31;

== matlab function m03/GiF/G/MATLAB Function1 ==
  data: N1 input; y output; N2 input; N3 input; J11 input; J21 input; J31 input
function y = fcn(N1, N2, N3, J11, J21, J31)

y = N1*J11+N2*J21+N3*J31;

== matlab function m03/GiF/G/MATLAB Function2 ==
  data: B1 input; y output; B2 input; B3 input; J11 input; J21 input; J31 input
function y = fcn(B1, B2, B3, J11, J21, J31)

y = B1*J11+B2*J21+B3*J31;

== matlab function m03/GiF/G/MATLAB Function3 ==
  data: T1 input; y output; T2 input; T3 input; J12 input; J22 input; J32 input
function y = fcn(T1, T2, T3, J12, J22, J32)

y = T1*J12+T2*J22+T3*J32;

== matlab function m03/GiF/G/MATLAB Function4 ==
  data: T1 input; y output; T2 input; T3 input; J13 input; J23 input; J33 input
function y = fcn(T1, T2, T3, J13, J23, J33)

y = T1*J13+T2*J23+T3*J33;

== matlab function m03/GiF/G/MATLAB Function5 ==
  data: N1 input; y output; N2 input; N3 input; J12 input; J22 input; J32 input
function y = fcn(N1, N2, N3, J12, J22, J32)

y = N1*J12+N2*J22+N3*J32;

== matlab function m03/GiF/G/MATLAB Function6 ==
  data: N1 input; y output; N2 input; N3 input; J13 input; J23 input; J33 input
function y = fcn(N1, N2, N3, J13, J23, J33)

y = N1*J13+N2*J23+N3*J33;

== matlab function m03/GiF/G/MATLAB Function7 ==
  data: B1 input; y output; B2 input; B3 input; J12 input; J22 input; J32 input
function y = fcn(B1, B2, B3, J12, J22, J32)

y = B1*J12+B2*J22+B3*J32;

== matlab function m03/GiF/G/MATLAB Function8 ==
  data: B1 input; y output; B2 input; B3 input; J13 input; J23 input; J33 input
function y = fcn(B1, B2, B3, J13, J23, J33)

y = B1*J13+B2*J23+B3*J33;

== matlab function m03/ODWR/DET ==
  data: a11 input; y output; a12 input; a13 input; a21 input; a22 input; a23 input; a31 input; a32 input; a33 input
function y = fcn(a11, a12, a13, a21, a22, a23, a31, a32, a33)

y = a11*a22*a33+a21*a32*a13+a31*a12*a23-a11*a32*a23-a31*a22*a13-a21*a12*a33;

== matlab function m03/ODWR/MATLAB Function ==
  data: a22 input; y output; a33 input; a23 input; a32 input; det input
function y = fcn(a22, a33, a23, a32, det)

y = (a22*a33-a23*a32)/det;

== matlab function m03/ODWR/MATLAB Function1 ==
  data: a12 input; a13 input; a32 input; y output; a33 input; det input
function y = fcn(a12, a13, a32, a33, det)

y = (a13*a32-a12*a33)/det;

== matlab function m03/ODWR/MATLAB Function2 ==
  data: a12 input; a13 input; a22 input; y output; a23 input; det input
function y = fcn(a12, a13, a22, a23, det)

y = (a12*a23-a13*a22)/det;

== matlab function m03/ODWR/MATLAB Function3 ==
  data: a21 input; a23 input; a31 input; y output; a33 input; det input
function y = fcn(a21, a23, a31, a33, det)

y = (a23*a31-a21*a33)/det;

== matlab function m03/ODWR/MATLAB Function4 ==
  data: a11 input; a13 input; a31 input; y output; a33 input; det input
function y = fcn(a11, a13, a31, a33, det)

y = (a11*a33-a13*a31)/det;

== matlab function m03/ODWR/MATLAB Function5 ==
  data: a11 input; y output; a13 input; a21 input; a23 input; det input
function y = fcn(a11, a13, a21, a23, det)

y = (a13*a21-a11*a23)/det;

== matlab function m03/ODWR/MATLAB Function6 ==
  data: a21 input; a22 input; y output; a31 input; a32 input; det input
function y = fcn(a21, a22, a31, a32, det)

y = (a21*a32-a22*a31)/det;

== matlab function m03/ODWR/MATLAB Function7 ==
  data: a11 input; y output; a12 input; a31 input; a32 input; det input
function y = fcn(a11, a12, a31, a32, det)

y = (a12*a31-a11*a32)/det;

== matlab function m03/ODWR/MATLAB Function8 ==
  data: a11 input; a12 input; a21 input; a22 input; y output; det input
function y = fcn(a11, a12, a21, a22, det)

y = (a11*a22-a12*a21)/det;

== matlab function m03/Kinematyka/MATLAB Function ==
  data: q1 input; y output; q3 input
function y = fcn(q1, q3)

y = (0.7 +0.5*cos(q3))*cos(q1);

== matlab function m03/Kinematyka/MATLAB Function1 ==
  data: q1 input; y output; q3 input
function y = fcn(q1, q3)

y = (0.7 +0.5*cos(q3))*sin(q1);

== matlab function m03/Kinematyka/MATLAB Function2 ==
  data: q2 input; y output; q3 input
function y = fcn(q2, q3)

y = q2+0.5*sin(q3);

== matlab function m03/Kinematyka/MATLAB Function3 ==
  data: q1 input; y output; q3 input
function y = fcn(q1, q3)

y = -sin(q1)*(0.7+0.5*cos(q3));

== matlab function m03/Kinematyka/MATLAB Function4 ==
  data: q1 input; y output; q3 input
function y = fcn(q1, q3)

y = -cos(q1)*0.5*sin(q3);

== matlab function m03/Kinematyka/MATLAB Function5 ==
  data: q1 input; y output; q3 input
function y = fcn(q1, q3)

y = cos(q1)*(0.7+0.5*cos(q3));

== matlab function m03/Kinematyka/MATLAB Function6 ==
  data: q1 input; y output; q3 input
function y = fcn(q1, q3)

y = -sin(q1)*0.5*sin(q3);

== matlab function m03/Kinematyka/MATLAB Function7 ==
  data: y output; q3 input
function y = fcn(q3)

y = 0.5*cos(q3);

== matlab function m03/RTR/Dynamika/C/MATLAB Function ==
  data: q3 input; y output; qp3 input
function y = fcn(q3, qp3)
%#codegen

y =qp3*(-0.6*sin(q3)-(4/15)*sin(q3)*cos(q3));

== matlab function m03/RTR/Dynamika/C/MATLAB Function1 ==
  data: qp1 input; y output; q3 input
function y = fcn(qp1,q3)
%#codegen

y = -qp1*(0.6*sin(q3)+(4/15)*sin(q3)*cos(q3));

== matlab function m03/RTR/Dynamika/C/MATLAB Function2 ==
  data: q3 input; y output; qp3 input
function y = fcn(q3, qp3)
%#codegen

y = -qp3*0.6*sin(q3);

== matlab function m03/RTR/Dynamika/C/MATLAB Function3 ==
  data: q3 input; y output; qp1 input
function y = fcn(q3, qp1)
%#codegen

y = qp1*(0.6*sin(q3)+(4/15)*sin(q3)*cos(q3));

== matlab function m03/RTR/Dynamika/D/MATLAB Function ==
  data: q3 input; y output
function y = fcn(q3)
%#codegen

y = 0.5*9.81*20*0.2*cos(q3);

== matlab function m03/RTR/Dynamika/F/MATLAB Function1 ==
  data: m11 input; y output
function y = fcn(m11)
%#codegen

y = 1/m11;

== matlab function m03/RTR/Dynamika/F/MATLAB Function2 ==
  data: m22 input; m23 input; y output; m32 input; m33 input
function y = fcn(m22, m23, m32, m33)
%#codegen

y = m33/(m22*m33-m23*m32);

== matlab function m03/RTR/Dynamika/F/MATLAB Function3 ==
  data: m22 input; m23 input; y output; m32 input; m33 input
function y = fcn(m22, m23, m32, m33)
%#codegen

y = -m32/(m22*m33-m23*m32);

== matlab function m03/RTR/Dynamika/F/MATLAB Function4 ==
  data: m22 input; m23 input; y output; m32 input; m33 input
function y = fcn(m22, m23, m32, m33)
%#codegen

y = -m23/(m22*m33-m23*m32);

== matlab function m03/RTR/Dynamika/F/MATLAB Function5 ==
  data: m22 input; m23 input; y output; m32 input; m33 input
function y = fcn(m22, m23, m32, m33)
%#codegen

y = m22/(m22*m33-m23*m32);

== matlab function m03/RTR/Dynamika/M/MATLAB Function ==
  data: u input; y output
function y = fcn(u)
%#codegen

y = 0.6 +1.8+(4/15)*(cos(u)*cos(u))+1.2*cos(u);

== matlab function m03/RTR/Dynamika/M/MATLAB Function2 ==
  data: u input; y output
function y = fcn(u)
%#codegen

y = 0.6*cos(u);

== matlab function m03/RTR/Dynamika/M/MATLAB Function3 ==
  data: u input; y output
function y = fcn(u)
%#codegen

y = 0.6*cos(u);
